simulink subsystem "PD_Long"  (R2022b)
settings: Solver=VariableStepAuto  StartTime=0.0  StopTime=10.0  RelTol=1e-3
settings Model: Creator=User  LastModifiedBy=User

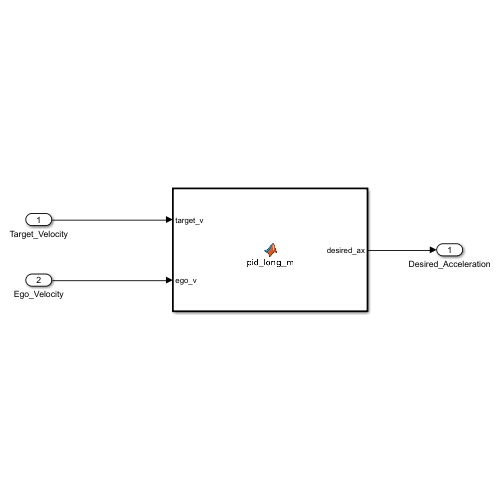
[thumbnail: Simulink's stored preview of the top-level diagram]
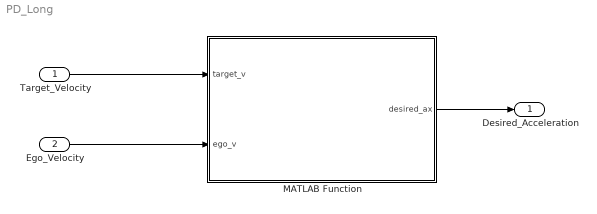
== system PD_Long ==
  Target_Velocity : Inport
  Ego_Velocity : Inport  Port=2
  MATLAB Function : MATLAB Function  TreatAsAtomicUnit=on
  Desired_Acceleration : Outport
  wires:
  Target_Velocity/1 -> MATLAB Function/1(target_v)
  Ego_Velocity/1 -> MATLAB Function/2(ego_v)
  MATLAB Function/1(desired_ax) -> Desired_Acceleration/1

== matlab function PD_Long/MATLAB Function ==
  data: target_v input; desired_ax output; ego_v input
function desired_ax = pid_long_m(target_v, ego_v)
    desired_ax = pid_long(target_v, ego_v);
    
end
